simulink model "euler"  (R2016a)
settings: Solver=VariableStepAuto  StartTime=0.0  StopTime=10  RelTol=1e-3
values from neighbouring files (symbols this model uses):
  hwx = 0    [TestFornonlineom.m]    (also in nonlineom.m = str2double(get(hObject,'String')))
  hwy = 0    [TestFornonlineom.m]    (also in nonlineom.m = str2double(get(hObject,'String')))
  hwz = 1000    [TestFornonlineom.m]    (also in nonlineom.m = str2double(get(hObject,'String')))
  Ix = 40    [TestForlineom.m]    (also in TestFornonlineom.m = 30; lineom.m = str2double(get(hObject,'String')); nonlineom.m = str2double(get(hObject,'String')))
  Iy = 50    [TestForlineom.m]    (also in TestFornonlineom.m = 40; lineom.m = str2double(get(hObject,'String')); nonlineom.m = str2double(get(hObject,'String')))
  Iz = 30    [TestForlineom.m]    (also in TestFornonlineom.m = 50; lineom.m = str2double(get(hObject,'String')); nonlineom.m = str2double(get(hObject,'String')))
  phi = 0    [TestForlineom.m]    (also in TestFornonlineom.m = 1.57079632679; lineom.m = str2num(get(hObject,'String')); nonlineom.m = str2num(get(hObject,'String')))
  psi = 0    [TestForlineom.m]    (also in TestFornonlineom.m = 1.57079632679; lineom.m = str2num(get(hObject,'String')); nonlineom.m = str2num(get(hObject,'String')))
  theta = 0.2    [TestForlineom.m]    (also in TestFornonlineom.m = 1.57079632679; lineom.m = str2num(get(hObject,'String')); nonlineom.m = str2num(get(hObject,'String')); saeroanim.m = (360/2/num:360/num:(360+360/2/num))*pi/180)
  w1 = 0.3    [TestFornonlineom.m]    (also in nonlineom.m = str2double(get(hObject,'String')))
  w2 = 0    [TestFornonlineom.m]    (also in nonlineom.m = str2double(get(hObject,'String')))
  w3 = 10    [TestFornonlineom.m]    (also in nonlineom.m = str2double(get(hObject,'String')))
libraries: aerolibanim x1, aerolibutil x1
settings Model: Creator=normal  LastModifiedBy=shrfm
settings DataIOCC: LimitDataPoints=on
settings DebuggingCC: AllowSymbolicDim=off
settings ModelReferenceCC: PropagateSignalLabelsOutOfModel=off
settings GRTTargetCC: GeneratePreprocessorConditionals=Use local settings

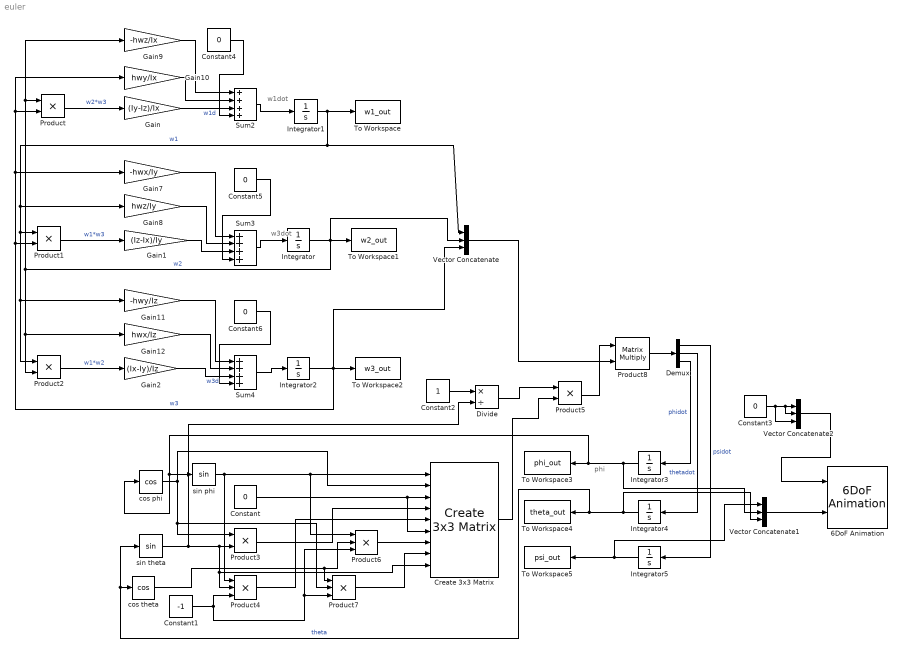
== system euler ==
  note: w3dot
  note: w1dot
  note: phi
  6DoF Animation : aerolibanim/6DoF Animation  u1=[0 4000 -2000 2000 -5000 -3000]  u2=0.01  u3=200  u4=[4000 0 -5000]  u5=Fixed position  u6=[2000 500 -3150]  u7=10  u8=on
  Constant{,3..6} (5 alike) : Constant  Value=0
  Constant1 : Constant  Value=-1
  Constant2 : Constant
  Create 3x3 Matrix : aerolibutil/Create 3x3 Matrix
  Demux : Demux  Outputs=3
  Divide : Product  Inputs=*/
  Gain : Gain  Gain=(Iy-Iz)/Ix
  Gain1 : Gain  Gain=(Iz-Ix)/Iy
  Gain10 : Gain  Gain=hwy/Ix
  Gain11 : Gain  Gain=-hwy/Iz
  Gain12 : Gain  Gain=hwx/Iz
  Gain2 : Gain  Gain=(Ix-Iy)/Iz
  Gain7 : Gain  Gain=-hwx/Iy
  Gain8 : Gain  Gain=hwz/Iy
  Gain9 : Gain  Gain=-hwz/Ix
  Integrator : Integrator  InitialCondition=w2
  Integrator1 : Integrator  InitialCondition=w1
  Integrator2 : Integrator  InitialCondition=w3
  Integrator3 : Integrator  InitialCondition=phi
  Integrator4 : Integrator  InitialCondition=theta
  Integrator5 : Integrator  InitialCondition=psi
  Product{,1..3,5} (5 alike) : Product
  Product4 : Product  Inputs=3
  Product6 : Product  Inputs=3
  Product7 : Product  Inputs=3
  Product8 : Product  Multiplication=Matrix(*)
  Sum2 : Sum  Inputs=4
  Sum3 : Sum  Inputs=4
  Sum4 : Sum  Inputs=4
  To Workspace : ToWorkspace  VariableName=w1_out  SaveFormat=Timeseries  SampleTime=-1
  To Workspace1 : ToWorkspace  VariableName=w2_out  SaveFormat=Timeseries  SampleTime=-1
  To Workspace2 : ToWorkspace  VariableName=w3_out  SaveFormat=Timeseries  SampleTime=-1
  To Workspace3 : ToWorkspace  VariableName=phi_out  SaveFormat=Timeseries  SampleTime=-1
  To Workspace4 : ToWorkspace  VariableName=theta_out  SaveFormat=Timeseries  SampleTime=-1
  To Workspace5 : ToWorkspace  VariableName=psi_out  SaveFormat=Timeseries  SampleTime=-1
  Vector Concatenate : Concatenate  NumInputs=3
  Vector Concatenate1 : Concatenate  NumInputs=3
  Vector Concatenate2 : Concatenate  NumInputs=3
  cos phi : Trigonometry  Operator=cos
  cos theta : Trigonometry  Operator=cos
  sin phi : Trigonometry
  sin theta : Trigonometry
  wires:
  Integrator1/1 -> To Workspace/1, Vector Concatenate/1, Gain8/1, Gain11/1, Product2/1, Product1/1  "w1"
  Integrator/1 -> Vector Concatenate/2, To Workspace1/1, Gain12/1, Product2/2, Gain9/1, Product/1  "w2"
  Integrator2/1 -> Vector Concatenate/3, To Workspace2/1, Product1/2, Gain7/1, Gain10/1, Product/2  "w3"
  Product/1 -> Gain/1  "w2*w3"
  Product1/1 -> Gain1/1  "w1*w3"
  Product2/1 -> Gain2/1  "w1*w2"
  sin phi/1 -> Product4/1, Product6/1, Create 3x3 Matrix/1
  cos phi/1 -> Product7/2, Product3/1, Create 3x3 Matrix/2
  Constant/1 -> Create 3x3 Matrix/6, Create 3x3 Matrix/3
  sin theta/1 -> Divide/2, Create 3x3 Matrix/9, Product4/2, Product3/2
  Product3/1 -> Create 3x3 Matrix/4
  Constant1/1 -> Product4/3, Product7/3, Product6/3
  Product4/1 -> Create 3x3 Matrix/5
  cos theta/1 -> Product7/1, Product6/2
  Product6/1 -> Create 3x3 Matrix/7
  Product7/1 -> Create 3x3 Matrix/8
  Constant2/1 -> Divide/1
  Divide/1 -> Product5/1
  Create 3x3 Matrix/1 -> Product5/2
  Product8/1 -> Demux/1
  Integrator3/1 -> Vector Concatenate1/2, cos phi/1, sin phi/1, To Workspace3/1
  Integrator4/1 -> Vector Concatenate1/3, To Workspace4/1, cos theta/1, sin theta/1  "theta"
  Product5/1 -> Product8/1
  Vector Concatenate/1 -> Product8/2
  Vector Concatenate2/1 -> 6DoF Animation/1
  Constant3/1 -> Vector Concatenate2/3, Vector Concatenate2/2, Vector Concatenate2/1
  Demux/3 -> Integrator3/1  "phidot"
  Demux/2 -> Integrator4/1  "thetadot"
  Demux/1 -> Integrator5/1  "psidot"
  Vector Concatenate1/1 -> 6DoF Animation/2
  Gain1/1 -> Sum3/3
  Sum3/1 -> Integrator/1
  Gain8/1 -> Sum3/2
  Gain7/1 -> Sum3/1
  Sum4/1 -> Integrator2/1
  Gain2/1 -> Sum4/3  "w3d"
  Gain12/1 -> Sum4/2
  Gain11/1 -> Sum4/1
  Integrator5/1 -> To Workspace5/1, Vector Concatenate1/1
  Gain/1 -> Sum2/3  "w1d"
  Gain10/1 -> Sum2/2
  Gain9/1 -> Sum2/1
  Sum2/1 -> Integrator1/1
  Constant4/1 -> Sum2/4
  Constant5/1 -> Sum3/4
  Constant6/1 -> Sum4/4
